simulink model "CAN_EthernetNetwork"  (R2019a)
settings: Solver=VariableStepAuto  StartTime=0.0  StopTime=100  FixedStep=0.003  RelTol=1e-3
libraries: truetime x9, cstblocks x2
settings Model: Creator=Alvaro UAO  LastModifiedBy=Alvaro UAO

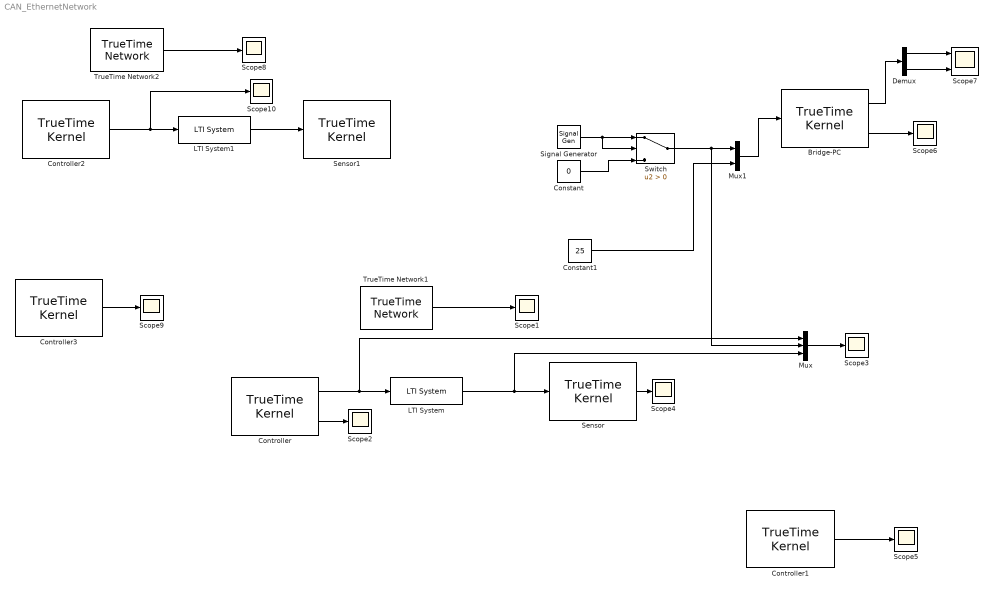
== system CAN_EthernetNetwork ==
  Bridge-PC : truetime/TrueTime Kernel  sfun=bridge_PC_init  args=[]  ninputsoutputs=[2 2]  ntriggers=0  trigtype=falling  nwnodenbr=[[1 3];[2 3]]  clockoffsetdrift=[0 0]  schedoutput=on  battery=off  poweroutput=off  label=1: 3\n2: 3
  Constant : Constant  Value=0
  Constant1 : Constant  Value=25
  Controller : truetime/TrueTime Kernel  sfun=controllerCAN_init  args=[]  ninputsoutputs=[0 1]  ntriggers=0  trigtype=falling  nwnodenbr=[1 2]  clockoffsetdrift=[0 0]  schedoutput=on  battery=off  poweroutput=off  label=1: 2
  Controller1 : truetime/TrueTime Kernel  sfun=disturbance_init  args=[]  ninputsoutputs=[0 0]  ntriggers=0  trigtype=falling  nwnodenbr=[1 4]  clockoffsetdrift=[0 0]  schedoutput=on  battery=off  poweroutput=off  label=1: 4
  Controller2 : truetime/TrueTime Kernel  sfun=controllerPTAP_init  args=[]  ninputsoutputs=[0 1]  ntriggers=0  trigtype=falling  nwnodenbr=[2 2]  clockoffsetdrift=[0 0]  schedoutput=off  battery=off  poweroutput=off  label=2: 2
  Controller3 : truetime/TrueTime Kernel  sfun=disturbanceEthernet_init  args=[]  ninputsoutputs=[0 0]  ntriggers=0  trigtype=falling  nwnodenbr=[2 4]  clockoffsetdrift=[0 0]  schedoutput=on  battery=off  poweroutput=off  label=2: 4
  Demux : Demux  Outputs=2
  LTI System : cstblocks/LTI System  sys=Quanzer  IC=[]
  LTI System1 : cstblocks/LTI System  sys=PTAP  IC=[]
  Mux : Mux  Inputs=3
  Mux1 : Mux  Inputs=2
  Scope{1..6,8..10} (9 alike) : Scope
  Scope7 : Scope  NumInputPorts=2
  Sensor : truetime/TrueTime Kernel  sfun=sensorCAN_init  args=[]  ninputsoutputs=[1 0]  ntriggers=0  trigtype=falling  nwnodenbr=[1 1]  clockoffsetdrift=[0 0]  schedoutput=on  battery=off  poweroutput=off  label=1: 1
  Sensor1 : truetime/TrueTime Kernel  sfun=sensorPTAP_init  args=[]  ninputsoutputs=[1 0]  ntriggers=0  trigtype=falling  nwnodenbr=[2 1]  clockoffsetdrift=[0 0]  schedoutput=off  battery=off  poweroutput=off  label=2: 1
  Signal Generator : SignalGenerator  WaveForm=square  Amplitude=3  Frequency=0.2
  Switch : Switch  Criteria=u2 > Threshold
  TrueTime Network1 : truetime/TrueTime Network  nwtype=CSMA/AMP (CAN)  nwnbr=1  nnodes=4  rate=250000  minsize=44  lossprob=0  seed=0  bandwidths=[0.5 0.5]  slotsize=512  schedule=[1 1 2]  memsize=80000  buftype=Common buffer  overflow=Retransmit  dynSchedule=0  miniSlotSize=0  NIT=0  QSortMode=FIFO  sync=0  irtSchedule=0  nrtLength=0  nodeGraph=0  scheduleoutput=on
  TrueTime Network2 : truetime/TrueTime Network  nwtype=CSMA/CD (Ethernet)  nwnbr=2  nnodes=4  rate=10000000  minsize=44  lossprob=0  seed=0  bandwidths=[0.5 0.5]  slotsize=512  schedule=[1 1 2]  memsize=80000  buftype=Common buffer  overflow=Retransmit  dynSchedule=0  miniSlotSize=0  NIT=0  QSortMode=FIFO  sync=0  irtSchedule=0  nrtLength=0  nodeGraph=0  scheduleoutput=on
  wires:
  Controller/1 -> Mux/1, LTI System/1
  LTI System/1 -> Mux/3, Sensor/1
  TrueTime Network1/1 -> Scope1/1
  Controller/2 -> Scope2/1
  Sensor/1 -> Scope4/1
  Bridge-PC/2 -> Scope6/1
  Mux/1 -> Scope3/1
  Signal Generator/1 -> Switch/2, Switch/1
  Constant/1 -> Switch/3
  Switch/1 -> Mux1/1, Mux/2
  Controller1/1 -> Scope5/1
  Controller2/1 -> Scope10/1, LTI System1/1
  LTI System1/1 -> Sensor1/1
  Mux1/1 -> Bridge-PC/1
  Constant1/1 -> Mux1/2
  Bridge-PC/1 -> Demux/1
  Demux/2 -> Scope7/2
  Demux/1 -> Scope7/1
  Controller3/1 -> Scope9/1
  TrueTime Network2/1 -> Scope8/1
